simulink model "Simple_RC_Circuit"  (R2022b)
settings: Solver=VariableStepAuto  StartTime=0.0  StopTime=10.0  MaxStep=1e-3  RelTol=1e-3
values from neighbouring files (symbols this model uses):
  C = 1e-6    (= 1e-06)    [Simple_RC.m]
  R = 1e3    (= 1000)    [Simple_RC.m]
settings Model: Creator=NourAldin  LastModifiedBy=NourAldin

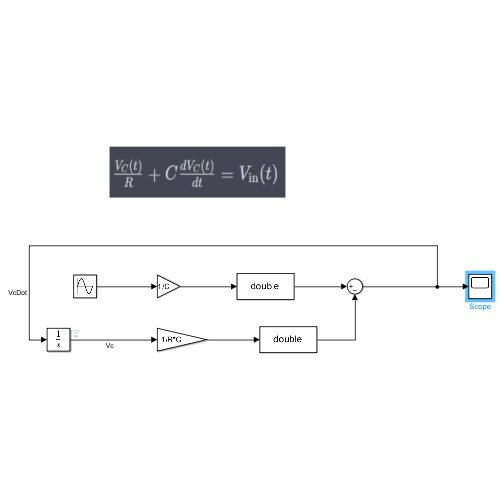
[thumbnail: Simulink's stored preview of the top-level diagram]
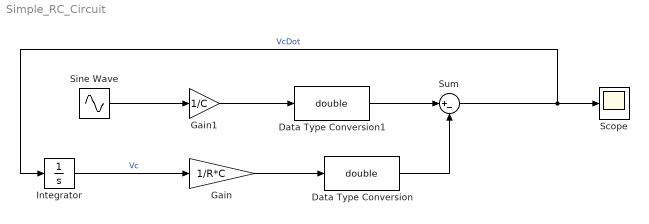
== system Simple_RC_Circuit ==
  Data Type Conversion : DataTypeConversion  OutDataTypeStr=double  SaturateOnIntegerOverflow=off  RndMeth=Floor
  Data Type Conversion1 : DataTypeConversion  OutDataTypeStr=double  SaturateOnIntegerOverflow=off  RndMeth=Floor
  Gain : Gain  Gain=1/R*C
  Gain1 : Gain  Gain=1/C
  Integrator : Integrator
  Scope : Scope
  Sine Wave : Sin  Amplitude=5  SampleTime=0
  Sum : Sum  Inputs=|+-
  wires:
  Sum/1 -> Scope/1, Integrator/1  "VcDot"
  Integrator/1 -> Gain/1  "Vc"
  Sine Wave/1 -> Gain1/1
  Gain/1 -> Data Type Conversion/1
  Gain1/1 -> Data Type Conversion1/1
  Data Type Conversion/1 -> Sum/2
  Data Type Conversion1/1 -> Sum/1
